simulink model "lab6"  (R2015b)
settings: Solver=ode45  SolverMode=SingleTasking  StartTime=0.0  StopTime=3  RelTol=1e-3
InitFcn:
  | clear functions
libraries: truetime x4
settings Model: Creator=peterfj  LastModifiedBy=andfro
settings DataIOCC: SaveFormat=Array
settings OptimizationCC: BlockReduction=off  BooleanDataType=off
settings DebuggingCC: SaveWithParameterizedLinksMsg=none  UnderspecifiedInitializationDetection=Classic  MergeDetectMultiDrivingBlocksExec=none  SignalResolutionControl=TryResolveAllWithWarning
settings HardwareCC: ProdBitPerPointer=32  ProdLargestAtomicFloat=None  ProdIntDivRoundTo=Undefined  ProdEndianess=Unspecified  ProdWordSize=32  ProdHWDeviceType=32-bit Generic  TargetUnknown=on
settings GRTTargetCC: GeneratePreprocessorConditionals=Disable all
settings ConfigComp: CovModelRefEnable=Off  CovSFcnEnable=off

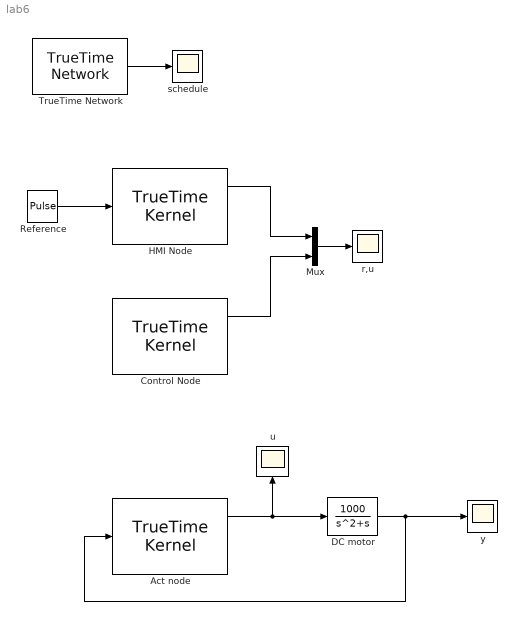
== system lab6 ==
  Act node : truetime/TrueTime Kernel  sfun=node_init_act  args=2  ninputsoutputs=[1 1]  ntriggers=0  trigtype=falling  nwnodenbr=[1 2]  clockoffsetdrift=[0 0]  schedoutput=on  battery=off  poweroutput=off  label=1: 2
  Control Node : truetime/TrueTime Kernel  sfun=node_init_control  args=2  ninputsoutputs=[1 1]  ntriggers=0  trigtype=falling  nwnodenbr=[1 3]  clockoffsetdrift=[0 0]  schedoutput=on  battery=off  poweroutput=off  label=1: 3
  "DC motor " : TransferFcn  Numerator=[1000]  Denominator=[1 1 0]
  HMI Node : truetime/TrueTime Kernel  sfun=node_init_hmi  args=2  ninputsoutputs=[1 1]  ntriggers=0  trigtype=falling  nwnodenbr=[1 1]  clockoffsetdrift=[0 0]  schedoutput=on  battery=off  poweroutput=off  label=1: 1
  Mux : Mux  Inputs=2
  Reference : DiscretePulseGenerator  PulseType=Time based  Amplitude=2  Period=1  PulseWidth=50  PhaseDelay=0.1  SampleTime=0.005
  TrueTime Network : truetime/TrueTime Network  nwtype=CSMA/AMP (CAN)  nwnbr=1  nnodes=3  rate=80000  minsize=44  lossprob=0  seed=0  bandwidths=[0.5 0.5]  slotsize=512  schedule=[1 1 2]  memsize=80000  buftype=Common buffer  overflow=Retransmit  dynSchedule=0  miniSlotSize=0  NIT=0  QSortMode=FIFO  sync=0  irtSchedule=0  nrtLength=0  nodeGraph=0  scheduleoutput=on
  r,u : Scope
  schedule : Scope
  u : Scope
  y : Scope
  wires:
  Reference/1 -> HMI Node/1
  TrueTime Network/1 -> schedule/1
  Mux/1 -> r,u/1
  Control Node/1 -> Mux/2
  HMI Node/1 -> Mux/1
  Act node/1 -> "DC motor "/1, u/1
  "DC motor "/1 -> y/1, Act node/1
